simulink model "BioEthanolProduction"  (R2016a)
settings: Solver=FixedStepAuto  StartTime=0.0  StopTime=50  FixedStep=0.001  RelTol=1e-3
settings Model: Creator=ACER  LastModifiedBy=ACER

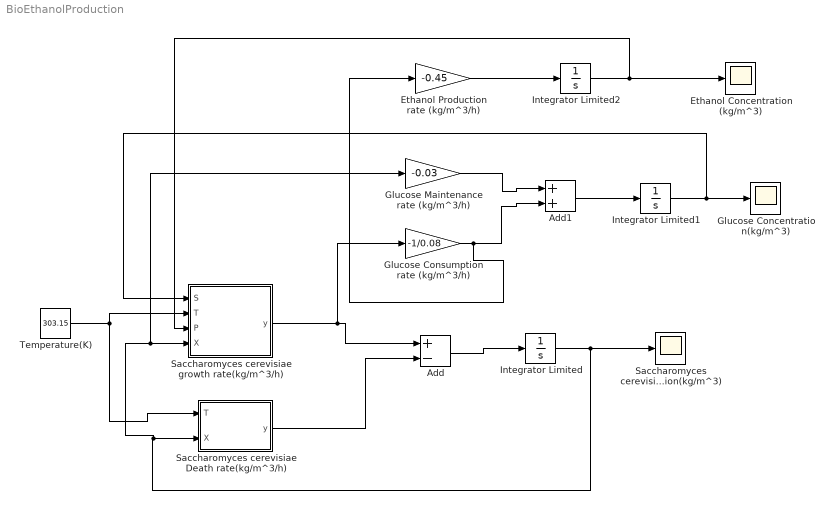
== system BioEthanolProduction ==
  Add : Sum  Inputs=+-
  Add1 : Sum
  Ethanol Concentration(kg/m^3) : Scope
  Ethanol Production rate (kg/m^3/h) : Gain  Gain=-0.45
  Glucose Concentration(kg/m^3) : Scope
  Glucose Consumption rate (kg/m^3/h) : Gain  Gain=-1/0.08
  Glucose Maintenance rate (kg/m^3/h) : Gain  Gain=-0.03
  Integrator Limited : Integrator  InitialCondition=1.5  LimitOutput=on  LowerSaturationLimit=0
  Integrator Limited1 : Integrator  InitialCondition=220  LimitOutput=on  LowerSaturationLimit=0
  Integrator Limited2 : Integrator  LimitOutput=on  UpperSaturationLimit=93  LowerSaturationLimit=0
  Saccharomyces cerevisiae Death rate(kg/m^3/h) : MATLAB Function  TreatAsAtomicUnit=on
  Saccharomyces cerevisiae Concentration(kg/m^3) : Scope
  Saccharomyces cerevisiae growth rate(kg/m^3/h) : MATLAB Function  TreatAsAtomicUnit=on
  Temperature(K) : Constant  Value=303.15
  wires:
  Temperature(K)/1 -> Saccharomyces cerevisiae Death rate(kg/m^3/h)/1(T), Saccharomyces cerevisiae growth rate(kg/m^3/h)/2(T)
  Saccharomyces cerevisiae growth rate(kg/m^3/h)/1(y) -> Glucose Consumption rate (kg/m^3/h)/1, Add/1
  Saccharomyces cerevisiae Death rate(kg/m^3/h)/1(y) -> Add/2
  Add/1 -> Integrator Limited/1
  Integrator Limited/1 -> Glucose Maintenance rate (kg/m^3/h)/1, Saccharomyces cerevisiae growth rate(kg/m^3/h)/4(X), Saccharomyces cerevisiae Death rate(kg/m^3/h)/2(X), Saccharomyces cerevisiae Concentration(kg/m^3)/1
  Glucose Maintenance rate (kg/m^3/h)/1 -> Add1/1
  Add1/1 -> Integrator Limited1/1
  Glucose Consumption rate (kg/m^3/h)/1 -> Ethanol Production rate (kg/m^3/h)/1, Add1/2
  Ethanol Production rate (kg/m^3/h)/1 -> Integrator Limited2/1
  Integrator Limited2/1 -> Saccharomyces cerevisiae growth rate(kg/m^3/h)/3(P), Ethanol Concentration(kg/m^3)/1
  Integrator Limited1/1 -> Saccharomyces cerevisiae growth rate(kg/m^3/h)/1(S), Glucose Concentration(kg/m^3)/1

== matlab function BioEthanolProduction/Saccharomyces cerevisiae Death rate(kg//m^3//h) ==
  data: T input; y output; X input
function y = fcn(T,X)
%#codegen

y = 1200000000*exp(-6860/T)*X;

== matlab function BioEthanolProduction/Saccharomyces cerevisiae growth rate(kg//m^3//h) ==
  data: S input; y output; T input; P input; X input
function y = fcn(S,T,P,X)
%#codegen

y = (0.33*exp(-((T-303)^2)/200)*S/(1.7+S))*((1-P/93)^0.52)*X;
